simulink model "ModelVerification"  (R2018b)
settings: Solver=VariableStepAuto  StartTime=0.0  StopTime=9e5  RelTol=1e-3
libraries: carnot x2, simulink x1
settings Model: Creator=manuel.koch  LastModifiedBy=manuel.koch

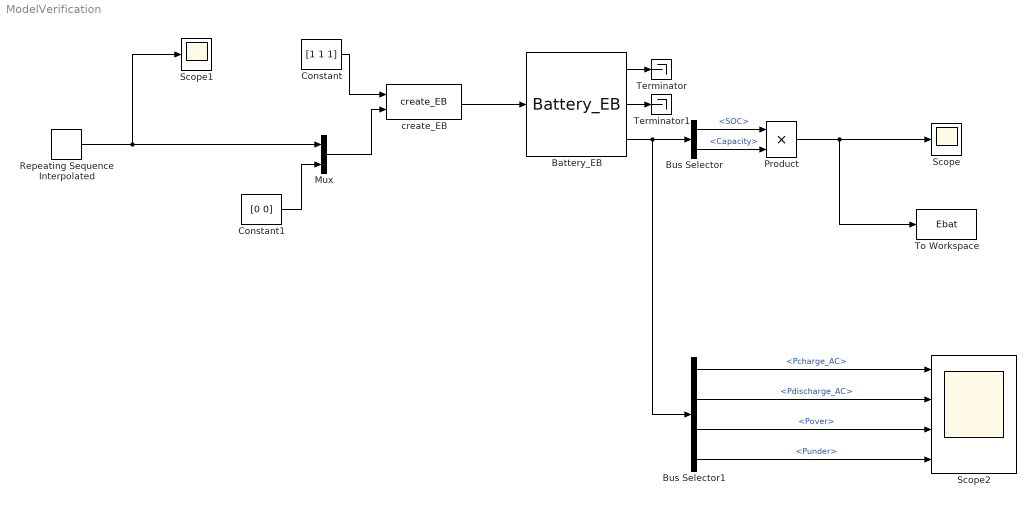
== system ModelVerification ==
  Battery_EB : carnot/Storage/Electric/Battery_EB  cap_kWh=5e6/3.6e6  eta_ch=0.9  eta_dis=0.9  cap0=1  SOC_max=1  SOC_min=0  Pmax=1000  Pmin=1000  P_standby=10
  Bus Selector : BusSelector  OutputSignals=SOC,Capacity
  Bus Selector1 : BusSelector  OutputSignals=Pcharge_AC,Pdischarge_AC,Pover,Punder
  Constant : Constant  Value=[1 1 1]
  Constant1 : Constant  Value=[0 0]
  Mux : Mux  Inputs=2
  Product : Product
  Repeating Sequence Interpolated : simulink/Sources/Repeating Sequence Interpolated  OutValues=[0 100 -100 10000 -10000 -10000]  TimeValues=[0 5e5 6e5 7e5 8e5 9e5]  LookUpMeth=Use Input Below  tsamp=1  OutMin=[]  OutMax=[]  OutDataTypeStr=double  OutputDataTypeScalingMode=double  OutDataType=fixdt(0,8)  OutScaling=2^-10
  Scope : Scope
  Scope1 : Scope
  Scope2 : Scope  NumInputPorts=4
  Terminator : Terminator
  Terminator1 : Terminator
  To Workspace : ToWorkspace  VariableName=Ebat  SaveFormat=Timeseries  SampleTime=-1
  create_EB : carnot/Source/Simple/create_EB  eID=Power only  f=50  pf1=1  pf2=1  pf3=1
  wires:
  create_EB/1 -> Battery_EB/1
  Constant/1 -> create_EB/1
  Battery_EB/3 -> Bus Selector1/1, Bus Selector/1
  Bus Selector/1 -> Product/1  "<SOC>"
  Bus Selector/2 -> Product/2  "<Capacity>"
  Battery_EB/1 -> Terminator/1
  Battery_EB/2 -> Terminator1/1
  Product/1 -> To Workspace/1, Scope/1
  Constant1/1 -> Mux/2
  Mux/1 -> create_EB/2
  Repeating Sequence Interpolated/1 -> Mux/1, Scope1/1
  Bus Selector1/1 -> Scope2/1  "<Pcharge_AC>"
  Bus Selector1/4 -> Scope2/4  "<Punder>"
  Bus Selector1/2 -> Scope2/2  "<Pdischarge_AC>"
  Bus Selector1/3 -> Scope2/3  "<Pover>"
